simulink model "quadcopter_package_delivery"  (R2025b)
settings: Solver=VariableStepAuto  StartTime=0.0  StopTime=timespot_spl(end)+2  FixedStep=0.01  MaxStep=1e-2  RelTol=1e-3  AbsTol=1e-3
model workspace (MATLAB code in the model file):
  | load('xy_data_membrane.mat');
undefined symbols (not defined in the file): air_rho, battery_capacity, filtD_altitude, filtD_attitude, filtD_motor, filtD_position, filtD_yaw, filtM_altitude, filtM_attitude, filtM_position, filtM_yaw, filtSpd_motor, kd_altitude, kd_attitude, kd_motor, kd_position, kd_yaw, ki_altitude, ki_attitude, ki_motor, ki_position, ki_yaw, kp_altitude, kp_attitude, kp_motor, kp_position, kp_yaw, limit_altitude, limit_attitude, limit_motor, limit_yaw, pkgDensity, pkgSize, planedepth, pos2attitude, propeller, qc_motor, qd_area, qd_drag, spline_data, spline_yaw, timespot_spl, waypoints, wind_speed, X, Y, Z
libraries: sm_lib x96, nesl_utility x42, fl_lib x21, slpidlib x13, ee_lib x9, octaquad_library x8, quadcopter_library x2, simulink x2, batteryecm_lib x1, sim3dlib x1, uavsim3dlib x1
(part 1 of 6)
CloseFcn:
  | try,close(h1_quadcopter_package_delivery),end
  | clear h1_quadcopter_package_delivery
  | try,close(h2_quadcopter_package_delivery),end
  | clear h2_quadcopter_package_delivery
  | try,close(h3_quadcopter_package_delivery),end
  | clear h3_quadcopter_package_delivery
  | try,close(h4_quadcopter_package_delivery),end
  | clear h4_quadcopter_package_delivery
Description:
  | Quadcopter Package Delivery
  | Copyright 2021-2025 The MathWorks, Inc.
settings Model: VariantFading=off  Creator=tianwang  LastModifiedBy=s400263
settings SolverCC: AutoScaleAbsTol=off  AlgebraicLoopSolver=TrustRegion  SolverResetMethod=Robust
settings DataIOCC: MaxDataPoints=10000  ReturnWorkspaceOutputs=off  SignalLoggingName=logsout_quadcopter_package_delivery
settings OptimizationCC: ReuseModelBlockBuffer=off
settings DebuggingCC: ParameterPrecisionLossMsg=none  UnconnectedInputMsg=warning  UnconnectedOutputMsg=warning  UnconnectedLineMsg=warning
settings ModelReferenceCC: EnableRefExpFcnMdlSchedulingChecks=on
settings SFSimCC: CustomCodeUndefinedFunction=UseInterfaceOnly
settings RTWCC: GPUComputeCapability=3.5  DLArmComputeVersion=19.05
settings SimscapeCC: ExplicitSolverDiagnosticOptions=none  SimscapeLogType=all  SimscapeLogSimulationStatistics=on  SimscapeLogToSDI=on  SimscapeLogName=simlog_quadcopter_package_delivery  SimscapeLogLimitData=off  SimscapeLogDataHistory=50000.0
settings DiagnosticsConfigSet: SimMechanicsConflictingReferenceFrames=none  SimMechanicsRigidlyBoundBlock=none
settings ExplorerConfigSet: SimMechanicsOpenEditorOnUpdate=off
settings ExplorerConfigSet: InternalSimMechanicsExplorerSettings=|
  | <ExplorerConfiguration>
  | 
  |   <canonicalview>default</canonicalview>
  | 
  |   <TilePanel>
  |     <TileInfo>
  |       <Tiles Columns="2" Count="4" Height="811" Rows="2" Width="1250">
  |         <Row Weight="0.485185"/>
  |         <Row Weight="0.514815"/>
  |         <Column Weight="0.566053"/>
  |         <Column Weight="0.433947"/>
  |         <Tile Height="1" Width="1" X="0" Y="0"/>
  |         <Tile Height="1" Width="1" X="0" Y="1"/>
  |         <Tile Height="1" Width="1" X="1" Y="0"/>
  |         <Tile Height="1" Width="1" X="1" Y="1"/>
  |       </Tiles>
  |     </TileInfo>
  |     <SceneInfo>
  |       <SceneViewer>
  |         <IsThisViewStd>
  |           <IsStandardView>off</IsStandardView>
  |           <StandardViewName>Front</StandardViewName>
  |         </IsThisViewStd>
  |         <BGColor>
  |           <R>1</R>
  |           <G>1</G>
  |           <B>1</B>
  |           <A>1</A>
  |         </BGColor>
  |         <Camera>
  |           <DoPerspective>off</DoPerspective>
  |           <Position>
  |             <X>25.203186982838027</X>
  |             <Y>-27.386918341389588</Y>
  |             <Z>37.998100145454515</Z>
  |           </Position>
  |           <Center>
  |             <X>0.97986640885492404</X>
  |             <Y>-1.3408869856974266</Y>
  |             <Z>3.3502290826120436</Z>
  |           </Center>
  |           <Up>
  |             <X>-0.49115478817381214</X>
  |             <Y>0.49587894163743207</Y>
  |             <Z>0.71615015834284224</Z>
  |           </Up>
  |           <XLim>3.6009022668466564</XLim>
  |           <YLim>3.6009022668466564</YLim>
  |           <ViewLimDist>0.01</ViewLimDist>
  |         </Camera>
  |       </SceneViewer>
  |       <SceneViewer>
  |         <IsThisViewStd>
  |           <IsStandardView>off</IsStandardView>
  |           <StandardViewName>Front</StandardViewName>
  |         </IsThisViewStd>
  |         <BGColor>
  |           <R>1</R>
  |           <G>1</G>
  |           <B>1</B>
  |           <A>1</A>
  |         </BGColor>
  |         <Camera>
  |           <DoPerspective>on</DoPerspective>
  |           <Position>
  |             <X>-2.0724459167642353</X>
  |             <Y>-1.9960352421392507</Y>
  |             <Z>4.1978106102606763</Z>
  |           </Position>
  |           <Center>
  |             <X>-2.0724459167642353</X>
  |             <Y>-1.9960352421392507</Y>
  |             <Z>3.1978106102606763</Z>
  |           </Center>
  |           <Up>
  |             <X>0</X>
  |             <Y>1</Y>
  |             <Z>0</Z>
  |           </Up>
  |           <XLim>0.46630765815499858</XLim>
  |           <YLim>0.46630765815499858</YLim>
  |           <ViewLimDist>0.01</ViewLimDist>
  |         </Camera>
  |       </SceneViewer>
  |       <SceneViewer>
  |         <IsThisViewStd>
  |           <IsStandardView>off</IsStandardView>
  |           <StandardViewName>Front</StandardViewName>
  |         </IsThisViewStd>
  |         <BGColor>
  |           <R>1</R>
  |           <G>1</G>
  |           <B>1</B>
  |           <A>1</A>
  |         </BGColor>
  |         <Camera>
  |           <DoPerspective>on</DoPerspective>
  |           <Position>
  |             <X>7</X>
  |             <Y>-2</Y>
  |             <Z>2</Z>
  |           </Position>
  |           <Center>
  |             <X>5</X>
  |             <Y>0</Y>
  |             <Z>0</Z>
  |           </Center>
  |           <Up>
  |             <X>-0.40824829046386313</X>
  |             <Y>0.40824829046386313</Y>
  |             <Z>0.81649658092772581</Z>
  |           </Up>
  |           <XLim>1.6153371117658344</XLim>
  |           <YLim>1.6153371117658344</YLim>
  |           <ViewLimDist>0.01</ViewLimDist>
  |         </Camera>
  |       </SceneViewer>
  |       <SceneViewer>
  |         <IsThisViewStd>
  |           <IsStandardView>off</IsStandardView>
  |           <StandardViewName>Front</StandardViewName>
  |         </IsThisViewStd>
  |         <BGColor>
  |           <R>1</R>
  |           <G>1</G>
  |           <B>1</B>
  |           <A>1</A>
  |         </BGColor>
  |         <Camera>
  |           <DoPerspective>on</DoPerspective>
  |           <Position>
  |             <X>-0.57244591676423529</X>
  |             <Y>-3.9960352421392509</Y>
  |             <Z>3.1978106102606763</Z>
  |           </Position>
  |           <Center>
  |             <X>-1.0409672024300534</X>
  |             <Y>-3.3713401945848265</Y>
  |             <Z>2.5731155627062519</Z>
  |           </Center>
  |           <Up>
  |             <X>-0.37481702853265453</X>
  |             <Y>0.49975603804353957</Y>
  |             <Z>0.78086880944303028</Z>
  |           </Up>
  |           <XLim>0.46630765815499858</XLim>
  |           <YLim>0.46630765815499858</YLim>
  |           <ViewLimDist>0.01</ViewLimDist>
  |         </Camera>
  |       </SceneViewer>
  |     </SceneInfo>
  |   </TilePanel>
  | 
  |   <MechEditorPanel>
  |     <GfxPanelCameraMap>
  |       <MapElement CameraMLId="Camera1" GfxPanelIndex="1"/>
  |       <MapElement CameraMLId="Camera5" GfxPanelIndex="2"/>
  |       <MapElement CameraMLId="Camera4" GfxPanelIndex="3"/>
  |     </GfxPanelCameraMap>
  |     <Cameras>
  |       <Camera>
  |         <Id>Camera1</Id>
  |         <Value>
  |           <Name>FixO Top</Name>
  |           <NativeCamera>
  |             <PositionTrackingFeature>Quadcopter.Camera.Cam_FixO_Top.R</PositionTrackingFeature>
  |             <CenterTrackingFeature>Quadcopter.Camera.Cam_FixO_Top.R</CenterTrackingFeature>
  |             <UpVectorTrackingFeature>Quadcopter.Camera.Cam_FixO_Top.R</UpVectorTrackingFeature>
  |             <CenterTrackingOrigin>off</CenterTrackingOrigin>
  |             <CenterTrackingDirection>+X</CenterTrackingDirection>
  |             <UpVectorTrackingDirection>+Y</UpVectorTrackingDirection>
  |           </NativeCamera>
  |         </Value>
  |       </Camera>
  |       <Camera>
  |         <Id>Camera2</Id>
  |         <Value>
  |           <Name>FixO L</Name>
  |           <NativeCamera>
  |             <PositionTrackingFeature>Quadcopter.Camera.Cam_FixO_L.R</PositionTrackingFeature>
  |             <CenterTrackingFeature>Quadcopter.Camera.Cam_FixO_L.R</CenterTrackingFeature>
  |             <UpVectorTrackingFeature>Quadcopter.Camera.Cam_FixO_L.R</UpVectorTrackingFeature>
  |             <CenterTrackingOrigin>off</CenterTrackingOrigin>
  |             <CenterTrackingDirection>+X</CenterTrackingDirection>
  |             <UpVectorTrackingDirection>+Z</UpVectorTrackingDirection>
  |           </NativeCamera>
  |         </Value>
  |       </Camera>
  |       <Camera>
  |         <Id>Camera3</Id>
  |         <Value>
  |           <Name>FixO F</Name>
  |           <NativeCamera>
  |             <PositionTrackingFeature>Quadcopter.Camera.Cam_FixO_F.R</PositionTrackingFeature>
  |             <CenterTrackingFeature>Quadcopter.Camera.Cam_FixO_F.R</CenterTrackingFeature>
  |             <UpVectorTrackingFeature>Quadcopter.Camera.Cam_FixO_F.R</UpVectorTrackingFeature>
  |             <CenterTrackingOrigin>off</CenterTrackingOrigin>
  |             <CenterTrackingDirection>+X</CenterTrackingDirection>
  |             <UpVectorTrackingDirection>+Z</UpVectorTrackingDirection>
  |           </NativeCamera>
  |         </Value>
  |       </Camera>
  |       <Camera>
  |         <Id>Camera4</Id>
  |         <Value>
  |           <Name>FixO UFL</Name>
  |           <NativeCamera>
  |             <PositionTrackingFeature>Quadcopter.Camera.Cam_FixO_UFL.R</PositionTrackingFeature>
  |             <CenterTrackingFeature>Quadcopter.Camera.Cam_FixO_UFL.R</CenterTrackingFeature>
  |             <UpVectorTrackingFeature>Quadcopter.Camera.Cam_FixO_UFL.R</UpVectorTrackingFeature>
  |             <CenterTrackingOrigin>off</CenterTrackingOrigin>
  |             <CenterTrackingDirection>+X</CenterTrackingDirection>
  |             <UpVectorTrackingDirection>+Z</UpVectorTrackingDirection>
  |           </NativeCamera>
  |         </Value>
  |       </Camera>
  |       <Camera>
  |         <Id>Camera5</Id>
  |         <Value>
  |           <Name>Track_Target</Name>
  |           <NativeCamera>
  |             <PositionTrackingFeature>Quadcopter.Camera.Cam_Target.R</PositionTrackingFeature>
  |             <CenterTrackingFeature>Quadcopter.Camera.Transform_Target.F</CenterTrackingFeature>
  |             <UpVectorTrackingFeature>Quadcopter.Camera.Transform_Target.F</UpVectorTrackingFeature>
  |             <CenterTrackingOrigin>on</CenterTrackingOrigin>
  |             <UpVectorTrackingDirection>+Z</UpVectorTrackingDirection>
  |           </NativeCamera>
  |         </Value>
  |       </Camera>
  |       <Camera>
  |         <Id>Camera6</Id>
  |         <Value>
  |           <Name>Track Body Forward</Name>
  |           <NativeCamera>
  |             <PositionTrackingFeature>Quadcopter.Body.Body.Cam_Body_Front.R</PositionTrackingFeature>
  |             <CenterTrackingFeature>Quadcopter.Body.Body.Cam_Body_Front.R</CenterTrackingFeature>
  |             <UpVectorTrackingFeature>Quadcopter.Body.Body.Cam_Body_Front.R</UpVectorTrackingFeature>
  |             <CenterTrackingOrigin>off</CenterTrackingOrigin>
  |             <CenterTrackingDirection>+X</CenterTrackingDirection>
  |             <UpVectorTrackingDirection>+Z</UpVectorTrackingDirection>
  |           </NativeCamera>
  |         </Value>
  |       </Camera>
  |     </Cameras>
  |     <VideoCreator>
  |       <IncludeTiles>All</IncludeTiles>
  |       <IncludeTime>on</IncludeTime>
  |       <IncludeWorldFrame>off</IncludeWorldFrame>
  |       <PlaybackSpeedRatio>1</PlaybackSpeedRatio>
  |       <FrameRate>60</FrameRate>
  |       <FrameSize>[1920, 1080]</FrameSize>
  |       <VideoFormat>UncompressedAVI</VideoFormat>
  |     </VideoCreator>
  |   </MechEditorPanel>
  | 
  |   <PlaybackSettings>
  |     <PlaybackSpeedFactor>4</PlaybackSpeedFactor>
  |   </PlaybackSettings>
  | 
  | </ExplorerConfiguration>

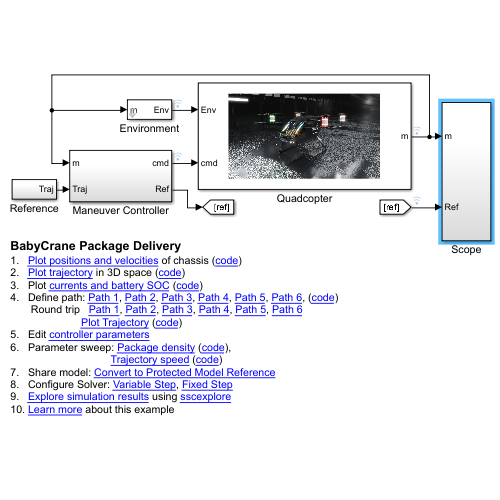
[thumbnail: Simulink's stored preview of the top-level diagram]
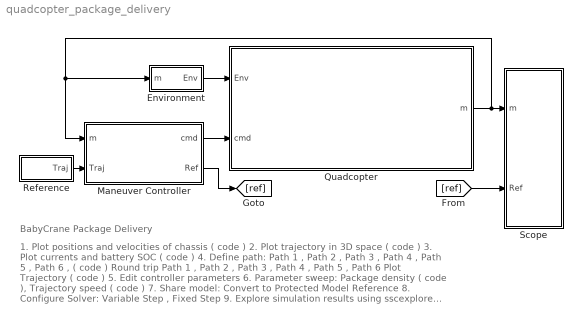
== system quadcopter_package_delivery ==
  note: BabyCrane Package Delivery
  note: 1. Plot positions and velocities of chassis ( code )
      | 2. Plot trajectory in 3D space ( code )
      | 3. Plot currents and battery SOC ( code )
      | 4. Define path: Path 1 , Path 2 , Path 3 , Path 4 , Path 5 , Path 6 , ( code )
      | Round trip Path 1 , Path 2 , Path 3 , Path 4 , Path 5 , Path 6
      | Plot Trajectory ( code )
      | 5. Edit controller parameters
      | 6. Parameter sweep: Package density ( code ),
      | Trajectory speed ( code )
      | 7. Share model: Convert to Protected Model Reference
      | 8. Configure Solver: Variable Step , Fixed Step
      | 9. Explore simulation results using sscexplore
      | 10. Learn more about this example
  Environment : Subsystem  mask{wind_speed_mag=wind_speed, height_max_wind=6, height_min_wind=2}
      mask prompts: wind_speed_mag "Wind Speed for Gust (m/s)"; height_max_wind "Lowest Height for Max Wind (m)"; height_min_wind "Maximum Height for Zero Wind (m)"
  Maneuver Controller : Subsystem
  Quadcopter : Subsystem
      mask Display: image('babyCrane.png', [0,0,0,0,80,80]);
  Reference : Subsystem
  Scope : Subsystem
  wires:
  Maneuver Controller/1(cmd) -> Quadcopter/2(cmd)
  Quadcopter/1(m) -> Maneuver Controller/1(m), Environment/1(m), Scope/1(m)
  Reference/1(Traj) -> Maneuver Controller/2(Traj)
  [ref] -> Scope/2(Ref)
  Maneuver Controller/2(Ref) -> [ref]
  Environment/1(Env) -> Quadcopter/1(Env)

== system quadcopter_package_delivery/Environment ==
  In Bus Element : Inport  PortName=m  Element=Chassis.pz
  Bias Height Min Wind : Bias  Bias=-height_min_wind  SaturateOnIntegerOverflow=off
  Bus Creator2 : BusCreator  Inputs=1
  Constant1 : Constant  Value=0
  Mux1 : Mux  Inputs=3
  Product1 : Product
  Pulse Generator2 : DiscretePulseGenerator  PulseType=Time based  Amplitude=wind_speed_mag  Period=10  PulseWidth=25  PhaseDelay=5
  Pulse Generator3 : DiscretePulseGenerator  PulseType=Time based  Amplitude=wind_speed_mag  Period=10  PulseWidth=25  PhaseDelay=9
  Saturation : Saturate  UpperLimit=height_max_wind-height_min_wind  LowerLimit=0  ZeroCross=off
  "Scale Wind by Height " : Gain  Gain=1/(height_max_wind-height_min_wind)
  Vec to Bus : Subsystem
  Env : Outport
  wires:
  In Bus Element/1 -> Bias Height Min Wind/1
  Bias Height Min Wind/1 -> Saturation/1
  Saturation/1 -> "Scale Wind by Height "/1
  "Scale Wind by Height "/1 -> Product1/1
  Constant1/1 -> Mux1/3  "vz"
  Pulse Generator3/1 -> Mux1/2  "vy"
  Pulse Generator2/1 -> Mux1/1  "vx"
  Mux1/1 -> Product1/2  "wind"
  Product1/1 -> Vec to Bus/1(V)  "wind"
  Vec to Bus/1(B) -> Bus Creator2/1
  Bus Creator2/1 -> Env/1  "Env"

== system quadcopter_package_delivery/Maneuver Controller ==
  In Bus Element13 : Inport  PortName=m
  In Bus Element3 : Inport  Port=2  PortName=Traj
  Altitude and YPR Control : Subsystem  mask{attitude_filtM=filtM_attitude, attitude_kp=kp_attitude, attitude_ki=ki_attitude, attitude_kd=kd_attitude, attitude_f=filtD_attitude, attitude_limit=limit_attitude, yaw_filtM=filtM_yaw, yaw_kp=kp_yaw, yaw_ki=ki_yaw, yaw_kd=kd_yaw, yaw_f=filtD_yaw, yaw_limit=limit_yaw, altitude_filtM=filtM_altitude, altitude_kp=kp_altitude, altitude_ki=ki_altitude, altitude_kd=kd_altitude, altitude_f=filtD_altitude, altitude_limit=limit_altitude}
      mask prompts: attitude_filtM "Filter Measurement (s)"; attitude_kp "Kp"; attitude_ki "Ki"; attitude_kd "Kd"; attitude_f "Derivative Filter Coefficient"; attitude_limit "Limit (m/s)"; yaw_filtM "Filter Measurement (s)"; yaw_kp "Kp"; yaw_ki "Ki"; yaw_kd "Kd"; yaw_f "Derivative Filter Coefficient"; yaw_limit "Limit (m/s)"; altitude_filtM "Filter Measurement (s)"; altitude_kp "Kp"; altitude_ki "Ki"; altitude_kd "Kd"; altitude_f "Derivative Filter Coefficient"; altitude_limit "Limit (m/s)"
      mask DialogControl Container3 Prompt: Attitude (Orientation)
      mask DialogControl Container4 Prompt: Yaw
      mask DialogControl Container_alt Prompt: Altitude (Orientation)
  Motor Mixer : Subsystem
  Position Control : Subsystem  mask{filt_pos4attitude=filtM_position, kp_xy2ypr=kp_position, ki_xy2ypr=ki_position, kd_xy2ypr=kd_position, filtD_xy2ypr=filtD_position, err2rp=pos2attitude}
      mask prompts: filt_pos4attitude "Filter Constant (s)"; kp_xy2ypr "Kp"; ki_xy2ypr "Ki"; kd_xy2ypr "Kd"; filtD_xy2ypr "Derivative Filter Coefficient"; err2rp "Position Error to Attitude"
  cmd : Outport
  Ref : Outport  Port=2
  wires:
  Motor Mixer/1(Cmd) -> cmd/1
  Altitude and YPR Control/2(Motor Roll) -> Motor Mixer/2(Roll Cmd)
  Altitude and YPR Control/1(Motor Pitch) -> Motor Mixer/1(Pitch Cmd)
  Altitude and YPR Control/3(Motor Yaw) -> Motor Mixer/3(Yaw Cmd)
  Altitude and YPR Control/4(Motor Thrust) -> Motor Mixer/4(Thrust Cmd)
  Position Control/2(Roll Cmd) -> Altitude and YPR Control/4(Roll Cmd)
  Position Control/1(Pitch Cmd) -> Altitude and YPR Control/3(Pitch Cmd)
  In Bus Element13/1 -> Position Control/1(m), Altitude and YPR Control/1(m)
  In Bus Element3/1 -> Position Control/2(Traj), Altitude and YPR Control/2(Ref)
  Position Control/3(Yaw Cmd) -> Altitude and YPR Control/5(Yaw Cmd)
  Position Control/4(Ref) -> Ref/1

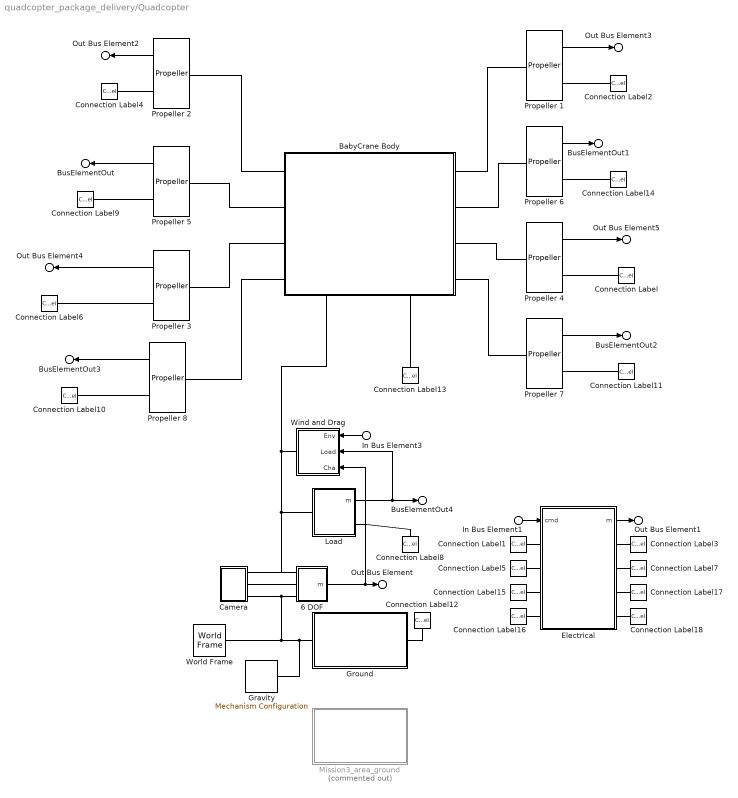
== system quadcopter_package_delivery/Quadcopter ==
  In Bus Element3 : Inport  PortName=Env  Element=wind
  In Bus Element1 : Inport  Port=2  PortName=cmd
  6 DOF : Subsystem
  BabyCrane Body : Subsystem
      settings: PortSchema="{\"entries\":[{\"content\":{\"sides\":[{\"content\":{\"connectorIds\":[\"LConn1\",\"LConn2\",\"LConn3\",\"LConn4\"]},\"type\":\"ConnectorPlacement.EquallySpacedRectSide\",\"uuid\":\"896afacf-a8ba-45b0-8fae-ae854689c003\"},{\"content\":{\"connectorIds\":[\"RConn1\",\"RConn2\",\"RConn3\",\"RConn4\"],\"side\":\"RIGHT\"},\"type\":\"ConnectorPlacement.EquallySpacedRectSide\",\"uuid\":\"d7f3e2ce-9a61-4f73-8b69-999e3aac03f1\"},{\"content\":{\"side\":\"TOP\"},\"type\":\"ConnectorPlacement.EquallySpacedRectSide\",\"uuid\":\"4926fabd-9420-42d5-af39-051dd107d6c5\"},{\"content\":{\"connectorIds\":[\"RConn5\",\"RConn6\"],\"side\":\"BOTTOM\"},\"type\":\"ConnectorPlacement.EquallySpacedRectSide\",\"uuid\":\"ae7c246a-1996-4b83-98e0-763fcfb4d202\"}]},\"type\":\"ConnectorPlacement.EquallySpacedConnector\",\"uuid\":\"d3b3fddd-7d8b-42c7-8e05-11f0e1d1d4f0\"}],\"packageUris\":[\"http://schema.mathworks.com/mf0/Connector/R2020b\"],\"version\":\"1.0\"}"
      mask Display: image('babycrane_chassis.png', [0,0,0,0,80,80]);
  Camera : Subsystem
  Connection Label : ConnectionLabel  Label=P4
  Connection Label1 : ConnectionLabel  Label=P4
  Connection Label10 : ConnectionLabel  Label=P8
  Connection Label11 : ConnectionLabel  Label=P7
  Connection Label12 : ConnectionLabel  Label=G
  Connection Label13 : ConnectionLabel  Label=G
  Connection Label14 : ConnectionLabel  Label=P6
  Connection Label15 : ConnectionLabel  Label=P6
  Connection Label16 : ConnectionLabel  Label=P8
  Connection Label17 : ConnectionLabel  Label=P5
  Connection Label18 : ConnectionLabel  Label=P7
  Connection Label2 : ConnectionLabel  Label=P1
  Connection Label3 : ConnectionLabel  Label=P1
  Connection Label4 : ConnectionLabel  Label=P2
  Connection Label5 : ConnectionLabel  Label=P2
  Connection Label6 : ConnectionLabel  Label=P3
  Connection Label7 : ConnectionLabel  Label=P3
  Connection Label8 : ConnectionLabel  Label=G
  Connection Label9 : ConnectionLabel  Label=P5
  Electrical : Subsystem  mask{trq_max=qc_motor.max_torque, power_max=qc_motor.max_power, trq_tc=qc_motor.time_const, eff_overall=qc_motor.efficiency, eff_spd=qc_motor.efficiency_spd, eff_trq=qc_motor.efficiency_trq, rotor_d=qc_motor.rotor_damping, kp=kp_motor, ki=ki_motor, kd=kd_motor, f_deriv=filtD_motor, f_spd=filtSpd_motor, max_trq_cmd=limit_motor}
      mask prompts: trq_max "Max Torque (N*m)"; power_max "Max Power (W)"; trq_tc "Time Constant, Torque (s)"; eff_overall "Efficiency (%)"; eff_spd "Speed for Efficiency (rpm)"; eff_trq "Torque for Efficiency (N*m)"; rotor_d "Rotor Damping (N*m/(rad/s))"; kp "Proportional"; ki "Integral"; kd "Derivative"; f_deriv "Filter on Error Derivative (N)"; f_spd "Filter on Speed Measurement (sec)"; max_trq_cmd "Saturation (N*m)"
      mask DialogControl Container4 Prompt: Motor
      mask DialogControl Container9 Prompt: Control
      mask Display: image('quadcopter_electric.png');
  Gravity : sm_lib/Utilities/Mechanism Configuration  UniformGravity=Constant  GravityVector=[0 0 -9.80665]  GravityVectorUnits=m/s^2  LinearizationDelta=0.001  JointModeTransitionNonlinearIterations=2
  Ground : Subsystem
      mask Display: image('ground_launch_target.PNG');
  Load : Subsystem
      mask Display:
      | %image('medical_kit.png');
      | image('load_package_basket.png');
  Mission3_area_ground : Subsystem  Commented=on
      mask Display: image('ground_launch_target.PNG');
  Propeller {1,3,5,7} (4 alike) : octaquad_library/Propeller  popup_prop_pos=CCW
  Propeller {2,4,6,8} (4 alike) : octaquad_library/Propeller  popup_prop_pos=CW
  Wind and Drag : Subsystem
  World Frame : sm_lib/Frames and Transforms/World Frame
  Out Bus Element : Outport  PortName=m  Element=Chassis
  Out Bus Element1 : Outport  PortName=m  Element=Motor
  Out Bus Element2 : Outport  PortName=m  Element=Prop2
  Out Bus Element3 : Outport  PortName=m  Element=Prop1
  Out Bus Element4 : Outport  PortName=m  Element=Prop3
  Out Bus Element5 : Outport  PortName=m  Element=Prop4
  BusElementOut : Outport  PortName=m  Element=Prop5
  BusElementOut1 : Outport  PortName=m  Element=Prop6
  BusElementOut2 : Outport  PortName=m  Element=Prop7
  BusElementOut3 : Outport  PortName=m  Element=Prop8
  BusElementOut4 : Outport  PortName=m  Element=Load
  wires:
  Propeller 4/1 -> Out Bus Element5/1
  Propeller 1/1 -> Out Bus Element3/1
  Propeller 3/1 -> Out Bus Element4/1
  Electrical/1(m) -> Out Bus Element1/1
  In Bus Element1/1 -> Electrical/1(cmd)
  Propeller 2/1 -> Out Bus Element2/1
  Propeller 5/1 -> BusElementOut/1
  Propeller 6/1 -> BusElementOut1/1
  Propeller 7/1 -> BusElementOut2/1
  Propeller 8/1 -> BusElementOut3/1
  6 DOF/1(m) -> Wind and Drag/3(Cha), Out Bus Element/1
  In Bus Element3/1 -> Wind and Drag/1(Env)
  Load/1(m) -> Wind and Drag/2(Load), BusElementOut4/1
  connections:
  Camera/RConn1 -- 6 DOF/LConn1 -- Load/LConn1 -- Wind and Drag/RConn1 -- BabyCrane Body/RConn5
  Connection Label/LConn1 -- Propeller 4/RConn1
  Connection Label2/LConn1 -- Propeller 1/RConn1
  Connection Label6/LConn1 -- Propeller 3/RConn1
  Gravity/RConn1 -- Ground/RConn1 -- Camera/RConn3 -- 6 DOF/LConn3 -- World Frame/RConn1
  Connection Label12/LConn1 -- Ground/LConn1
  Camera/RConn2 -- 6 DOF/LConn2
  Connection Label13/LConn1 -- BabyCrane Body/RConn6
  BabyCrane Body/RConn1 -- Propeller 1/LConn1
  BabyCrane Body/LConn1 -- Propeller 2/LConn1
  Connection Label4/LConn1 -- Propeller 2/RConn1
  Propeller 3/LConn1 -- BabyCrane Body/LConn3
  BabyCrane Body/RConn3 -- Propeller 4/LConn1
  BabyCrane Body/LConn2 -- Propeller 5/LConn1
  BabyCrane Body/RConn2 -- Propeller 6/LConn1
  BabyCrane Body/RConn4 -- Propeller 7/LConn1
  BabyCrane Body/LConn4 -- Propeller 8/LConn1
  Connection Label9/LConn1 -- Propeller 5/RConn1
  Connection Label10/LConn1 -- Propeller 8/RConn1
  Connection Label11/LConn1 -- Propeller 7/RConn1
  Connection Label14/LConn1 -- Propeller 6/RConn1
  Electrical/RConn1 -- Connection Label3/LConn1
  Connection Label7/LConn1 -- Electrical/RConn2
  Connection Label5/LConn1 -- Electrical/LConn2
  Connection Label1/LConn1 -- Electrical/LConn1
  Connection Label15/LConn1 -- Electrical/LConn3
  Connection Label16/LConn1 -- Electrical/LConn4
  Electrical/RConn3 -- Connection Label17/LConn1
  Electrical/RConn4 -- Connection Label18/LConn1
  Load/RConn1 -- Connection Label8/LConn1

== system quadcopter_package_delivery/Reference ==
  Clock1 : Clock
  Derivative : Subsystem
  Interpolate Spline Points : Subsystem
  Out Bus Element : Outport  PortName=Traj  Element=pos
  Out Bus Element1 : Outport  PortName=Traj  Element=vel
  Out Bus Element2 : Outport  PortName=Traj  Element=yaw
  wires:
  Clock1/1 -> Interpolate Spline Points/1(In1)
  Interpolate Spline Points/2(des_pos) -> Out Bus Element/1, Derivative/1(des xyz)
  Interpolate Spline Points/1(Yaw) -> Out Bus Element2/1
  Derivative/1(des_vel) -> Out Bus Element1/1

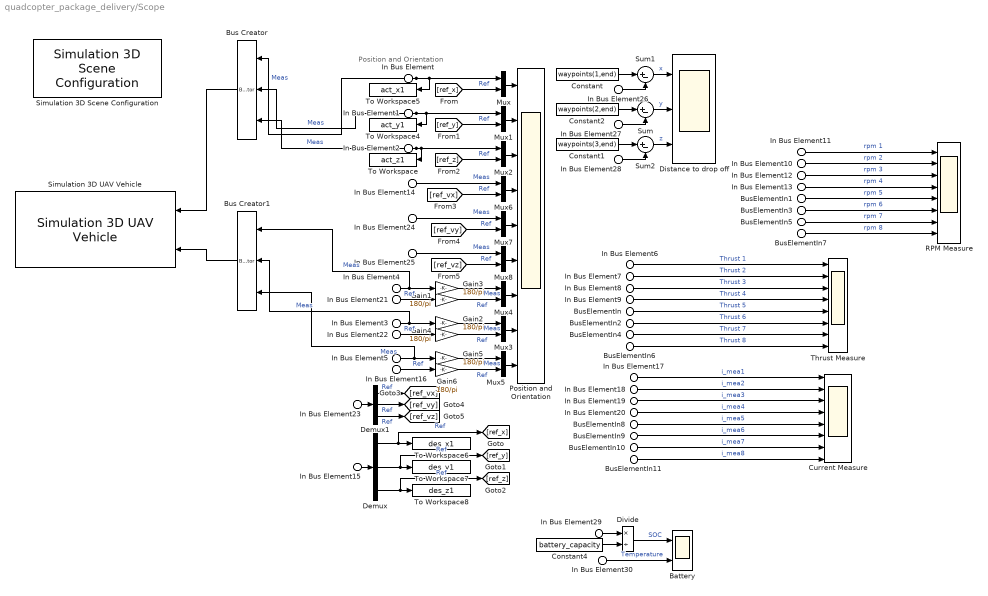
== system quadcopter_package_delivery/Scope ==
  note: Position and Orientation
  In Bus Element : Inport  PortName=m  Element=Chassis.px
  In Bus Element26 : Inport  PortName=m  Element=Chassis.px
  In Bus Element1 : Inport  PortName=m  Element=Chassis.py
  In Bus Element27 : Inport  PortName=m  Element=Chassis.py
  In Bus Element2 : Inport  PortName=m  Element=Chassis.pz
  In Bus Element28 : Inport  PortName=m  Element=Chassis.pz
  In Bus Element3 : Inport  PortName=m  Element=Chassis.pitch
  In Bus Element4 : Inport  PortName=m  Element=Chassis.roll
  In Bus Element5 : Inport  PortName=m  Element=Chassis.yaw
  In Bus Element14 : Inport  PortName=m  Element=Chassis.vx
  In Bus Element24 : Inport  PortName=m  Element=Chassis.vy
  In Bus Element25 : Inport  PortName=m  Element=Chassis.vz
  In Bus Element7 : Inport  PortName=m  Element=Prop2.thrust
  In Bus Element10 : Inport  PortName=m  Element=Prop2.w
  In Bus Element6 : Inport  PortName=m  Element=Prop1.thrust
  In Bus Element11 : Inport  PortName=m  Element=Prop1.w
  In Bus Element8 : Inport  PortName=m  Element=Prop3.thrust
  In Bus Element12 : Inport  PortName=m  Element=Prop3.w
  In Bus Element9 : Inport  PortName=m  Element=Prop4.thrust
  In Bus Element13 : Inport  PortName=m  Element=Prop4.w
  In Bus Element17 : Inport  PortName=m  Element=Motor.Mot1.i
  In Bus Element18 : Inport  PortName=m  Element=Motor.Mot2.i
  In Bus Element19 : Inport  PortName=m  Element=Motor.Mot3.i
  In Bus Element20 : Inport  PortName=m  Element=Motor.Mot4.i
  In Bus Element29 : Inport  PortName=m  Element=Motor.Battery.SOC
  In Bus Element30 : Inport  PortName=m  Element=Motor.Battery.degC
  BusElementIn8 : Inport  PortName=m  Element=Motor.Mot5.i
  BusElementIn9 : Inport  PortName=m  Element=Motor.Mot6.i
  BusElementIn10 : Inport  PortName=m  Element=Motor.Mot7.i
  BusElementIn11 : Inport  PortName=m  Element=Motor.Mot8.i
  BusElementIn : Inport  PortName=m  Element=Prop5.thrust
  BusElementIn1 : Inport  PortName=m  Element=Prop5.w
  BusElementIn2 : Inport  PortName=m  Element=Prop6.thrust
  BusElementIn3 : Inport  PortName=m  Element=Prop6.w
  BusElementIn4 : Inport  PortName=m  Element=Prop7.thrust
  BusElementIn5 : Inport  PortName=m  Element=Prop7.w
  BusElementIn6 : Inport  PortName=m  Element=Prop8.thrust
  BusElementIn7 : Inport  PortName=m  Element=Prop8.w
  In Bus Element15 : Inport  Port=2  PortName=Ref  Element=pos
  In Bus Element16 : Inport  Port=2  PortName=Ref  Element=yaw
  In Bus Element21 : Inport  Port=2  PortName=Ref  Element=roll
  In Bus Element22 : Inport  Port=2  PortName=Ref  Element=pitch
  In Bus Element23 : Inport  Port=2  PortName=Ref  Element=vel
  Battery : Scope  NumInputPorts=2
      settings: ActiveDisplayYMinimum=0.99986924380899678  ActiveDisplayYMaximum=0.99998918514322743
  Bus Creator : BusCreator  Inputs=3
  Bus Creator1 : BusCreator  Inputs=3
  Constant : Constant  Value=waypoints(1,end)
  Constant1 : Constant  Value=waypoints(3,end)
  Constant2 : Constant  Value=waypoints(2,end)
  Constant4 : Constant  Value=battery_capacity
  Current Measure : Scope  NumInputPorts=8
      settings: ActiveDisplayYMinimum=-14.67068968845636  ActiveDisplayYMaximum=25.248658155303175  DataLoggingVariableName=ScopeData2
  Demux : Demux  Outputs=3
  Demux1 : Demux  Outputs=3
  Distance to drop off : Scope  NumInputPorts=3
      settings: ActiveDisplayYMinimum=-0.41336623089959534  ActiveDisplayYMaximum=8.0037382763618758
  Divide : Product  Inputs=*/
  Gain{1..6} (6 alike) : Gain  Gain=180/pi
  Mux{,1..8} (9 alike) : Mux  Inputs=2
  Position and Orientation : Scope  NumInputPorts=9
      settings: Title=px  ActiveDisplayYMinimum=-17.050493412525565  ActiveDisplayYMaximum=19.852943833755543  DataLoggingVariableName=ScopeData2
  RPM Measure : Scope  NumInputPorts=8
      settings: ActiveDisplayYMinimum=-4929.5215436676654  ActiveDisplayYMaximum=4929.5236910244057  DataLoggingVariableName=ScopeData2
  Simulation 3D Scene Configuration : sim3dlib/Simulation 3D Scene Configuration  Priority=0  ProjectFormat=Unreal Editor  SceneDesc=Airport  ProjectName=C:\Program Files\MATLAB\R2025b\toolbox\shared\sim3d_projects\automotive_project_windows\UE\WindowsNoEditor\VehicleSimulation.exe  ScenePath=/Game/Maps/HwStrght  UEProjPath=C:\Users\s400263\OneDrive - Cranfield University\Documents\Unreal Projects\GoAero_1\GoAero_1.uproject  EnableOpenDRIVE=off  vehTagList={'Custom';'Scene Origin';'SimulinkVehicle1'}  vehTag=SimulinkVehicle1  AttachedCameraRelativeTranslation=[0 0 0]  FreeCameraDefaultInitialTranslation=[-6, 0, 2]  AttachedCameraRelativeRotation=[0 0 0]  FreeCameraDefaultInitialRotation=[0, -15, 0]  ViewpointName=Custom  FreeCameraInitialTranslation=[-6, 0, 2]  ViewpointTranslation=[0 0 0]  FreeCameraInitialRotation=[0, -15, 0]  ViewpointRotation=[0 0 0]  OpVisEn=off  Ts=.02  EnableWindow=on  EnableRemoteAccess=off  EnableWeather=off  SunAzimuth=90  SunAltitude=40.0  EnableGeospatialSun=off  Latitude=0  Longitude=0  Date=2023-01-01  Time=10:30:00  GeoTimeZone=-5.0  SunDaylightSaving=off  wind=1  clouds=10  EnableVolumetricClouds=off  CloudCoverage=0  CloudAltitude=6  fog=0  rain=0  RaindropsEffect=off  SnowDensity=0  EnableGeospatial=off  TilesetSource=Earth terrain  UseTrueOrigin=off  OriginHeight=200  OriginLatitude=40.744652  OriginLongitude=-73.988864  MapStyle=Aerial  AdditionalAssetIDs=[]  UseAdvancedSunSky=off  SolarTime=11  TimeZone=-5  Day=21  Month=9  Year=2022  UseDaylightSavingTime=on  DSTStartDay=10  DSTStartMonth=3  DSTEndDay=3  DSTEndMonth=11  DSTSwitchHour=2  sensorTag=MainCamera1  sensorId=1  sensorName=MainCamera1  mountLoc=Origin  offsetFlag=off  tmountOffset=[0, 0, 0]  rmountOffset=[0, 0, 0]  HorizontalResolution=1280  VerticalResolution=720  HorizontalFOV=60  mountPoint=[0 0 0]  mountOrientation=[0 0 0]  aMode=0  ID=1  GeoTrigger=Inactive  ViewNameList={'Custom'}  ViewTranslationList={'[-6 0 2]'}  ViewRotationList={'[0 -15 0]'}
      settings: LibrarySourceBlock=aerolibsim3d/Simulation 3D Scene Configuration
  Simulation 3D UAV Vehicle : uavsim3dlib/Simulation 3D UAV Vehicle  Priority=-1  Mesh=Quadrotor  MeshPath=/MathWorksUAVContent/UAVs/HexaRotorUAV/HexaRotor.HexaRotor  Color=Black  ActorName=SimulinkVehicle1  UseGlobalFrame=off  InitialTranslation=[0 0 0]  InitialRotation=[0 0 0]  InitialTranslationGlobal=[0 0 0]  InitialGeoOrigin=[0 0 0]  InitialRotationGlobal=[0 0 0]  SampleTime=-1  ActorType=SimulinkVehicle  ID=1  aMode=4  ActorTag=SimulinkVehicle1
  Sum : Sum  Inputs=|+-
  Sum1 : Sum  Inputs=|+-
  Sum2 : Sum  Inputs=|+-
  Thrust Measure : Scope  NumInputPorts=8
      settings: ActiveDisplayString=4  ActiveDisplayYMinimum=-7.0248060598913291  ActiveDisplayYMaximum=63.22325453902198
  To Workspace : ToWorkspace  VariableName=act_z1  SampleTime=-1
  To Workspace4 : ToWorkspace  VariableName=act_y1  SampleTime=-1
  To Workspace5 : ToWorkspace  VariableName=act_x1  SampleTime=-1
  To Workspace6 : ToWorkspace  VariableName=des_x1  SampleTime=-1
  To Workspace7 : ToWorkspace  VariableName=des_y1  SampleTime=-1
  To Workspace8 : ToWorkspace  VariableName=des_z1  SampleTime=-1
  wires:
  In Bus Element7/1 -> Thrust Measure/2  "Thrust 2"
  In Bus Element9/1 -> Thrust Measure/4  "Thrust 4"
  In Bus Element8/1 -> Thrust Measure/3  "Thrust 3"
  In Bus Element6/1 -> Thrust Measure/1  "Thrust 1"
  In Bus Element11/1 -> RPM Measure/1  "rpm 1"
  In Bus Element10/1 -> RPM Measure/2  "rpm 2"
  In Bus Element12/1 -> RPM Measure/3  "rpm 3"
  In Bus Element13/1 -> RPM Measure/4  "rpm 4"
  Demux/3 -> [ref_z], To Workspace8/1  "Ref"
  In Bus Element2/1 -> Bus Creator/3, Mux2/1, To Workspace/1  "Meas"
  In Bus Element17/1 -> Current Measure/1  "i_mea1"
  In Bus Element18/1 -> Current Measure/2  "i_mea2"
  In Bus Element19/1 -> Current Measure/3  "i_mea3"
  In Bus Element20/1 -> Current Measure/4  "i_mea4"
  Gain2/1 -> Mux3/1  "Meas"
  Gain3/1 -> Mux4/1  "Meas"
  Gain5/1 -> Mux5/1  "Meas"
  Demux/2 -> [ref_y], To Workspace7/1  "Ref"
  In Bus Element1/1 -> Bus Creator/2, Mux1/1, To Workspace4/1  "Meas"
  Demux/1 -> To Workspace6/1, [ref_x]  "Ref"
  In Bus Element/1 -> Bus Creator/1, Mux/1, To Workspace5/1  "Meas"
  In Bus Element28/1 -> Sum2/2
  Constant1/1 -> Sum2/1
  Constant2/1 -> Sum/1
  In Bus Element27/1 -> Sum/2
  Constant/1 -> Sum1/1
  In Bus Element26/1 -> Sum1/2
  Sum/1 -> Distance to drop off/2  "y"
  Sum1/1 -> Distance to drop off/1  "x"
  Sum2/1 -> Distance to drop off/3  "z"
  Mux/1 -> Position and Orientation/1
  Mux1/1 -> Position and Orientation/2
  Mux2/1 -> Position and Orientation/3
  Mux3/1 -> Position and Orientation/8
  Mux4/1 -> Position and Orientation/7
  Mux5/1 -> Position and Orientation/9
  In Bus Element15/1 -> Demux/1
  [ref_x] -> Mux/2  "Ref"
  [ref_y] -> Mux1/2  "Ref"
  [ref_z] -> Mux2/2  "Ref"
  In Bus Element23/1 -> Demux1/1
  Demux1/1 -> [ref_vx]  "Ref"
  Demux1/2 -> [ref_vy]  "Ref"
  Demux1/3 -> [ref_vz]  "Ref"
  Mux8/1 -> Position and Orientation/6
  Mux7/1 -> Position and Orientation/5
  Mux6/1 -> Position and Orientation/4
  [ref_vx] -> Mux6/2  "Ref"
  [ref_vy] -> Mux7/2  "Ref"
  [ref_vz] -> Mux8/2  "Ref"
  In Bus Element14/1 -> Mux6/1  "Meas"
  In Bus Element24/1 -> Mux7/1  "Meas"
  In Bus Element25/1 -> Mux8/1  "Meas"
  In Bus Element21/1 -> Gain1/1  "Ref"
  In Bus Element22/1 -> Gain4/1  "Ref"
  In Bus Element16/1 -> Gain6/1  "Ref"
  In Bus Element4/1 -> Bus Creator1/1, Gain3/1  "Meas"
  Gain1/1 -> Mux4/2  "Ref"
  In Bus Element3/1 -> Bus Creator1/2, Gain2/1  "Meas"
  Gain4/1 -> Mux3/2  "Ref"
  In Bus Element5/1 -> Bus Creator1/3, Gain5/1  "Meas"
  Gain6/1 -> Mux5/2  "Ref"
  In Bus Element29/1 -> Divide/1
  Constant4/1 -> Divide/2
  Divide/1 -> Battery/1  "SOC"
  In Bus Element30/1 -> Battery/2  "Temperature"
  BusElementIn/1 -> Thrust Measure/5  "Thrust 5"
  BusElementIn2/1 -> Thrust Measure/6  "Thrust 6"
  BusElementIn4/1 -> Thrust Measure/7  "Thrust 7"
  BusElementIn6/1 -> Thrust Measure/8  "Thrust 8"
  BusElementIn1/1 -> RPM Measure/5  "rpm 5"
  BusElementIn3/1 -> RPM Measure/6  "rpm 6"
  BusElementIn5/1 -> RPM Measure/7  "rpm 7"
  BusElementIn7/1 -> RPM Measure/8  "rpm 8"
  BusElementIn8/1 -> Current Measure/5  "i_mea5"
  BusElementIn9/1 -> Current Measure/6  "i_mea6"
  BusElementIn10/1 -> Current Measure/7  "i_mea7"
  BusElementIn11/1 -> Current Measure/8  "i_mea8"
  Bus Creator/1 -> Simulation 3D UAV Vehicle/1
  Bus Creator1/1 -> Simulation 3D UAV Vehicle/2

== system quadcopter_package_delivery/Environment/Vec to Bus ==
  V : Inport
  Bus Creator : BusCreator  Inputs=3
  Demux : Demux  Outputs=3
  B : Outport
  wires:
  Demux/3 -> Bus Creator/3  "vz"
  V/1 -> Demux/1
  Demux/1 -> Bus Creator/1  "vx"
  Demux/2 -> Bus Creator/2  "vy"
  Bus Creator/1 -> B/1  "wind"
